simulink model "sf_abstemporal_basic"  (R2017b)
settings: Solver=FixedStepDiscrete  StartTime=0.0  StopTime=10.0  FixedStep=0.1  RelTol=1e-3  EnableMultiTasking=on
settings Model: Creator=The MathWorks, Inc.  LastModifiedBy=The MathWorks, Inc.
settings DataIOCC: LimitDataPoints=on  SaveFormat=Array
settings OptimizationCC: ExpressionDepthLimit=2147483647  LifeSpan=inf
settings DebuggingCC: UnderspecifiedInitializationDetection=Classic  MergeDetectMultiDrivingBlocksExec=none  SolverPrmCheckMsg=warning  FcnCallInpInsideContextMsg=warning  StateNameClashWarn=warning  StrictBusMsg=Warning  SFUnexpectedBacktrackingDiag=warning  SFNoUnconditionalDefaultTransitionDiag=warning  SFExecutionAtInitializationDiag=none
settings HardwareCC: ProdBitPerPointer=32  ProdBitPerSizeT=32  ProdBitPerPtrDiffT=32  ProdLargestAtomicFloat=None  ProdIntDivRoundTo=Undefined  ProdEndianess=Unspecified  ProdWordSize=32  ProdHWDeviceType=32-bit Generic
settings ModelReferenceCC: PropagateSignalLabelsOutOfModel=off
settings SFSimCC: SimParseCustomCode=off
settings CodeAppCC: StateflowObjectComments=on
settings GRTTargetCC: TargetLangStandard=C89/C90 (ANSI)  GeneratePreprocessorConditionals=Disable all  CombineOutputUpdateFcns=off  GRTInterface=on
settings ConfigComp: CovMetricSettings=dw  CovHtmlReporting=on  CovSaveCumulativeToWorkspaceVar=on  CovSaveSingleToWorkspaceVar=on  CovExternalEMLEnable=off  CovSFcnEnable=off

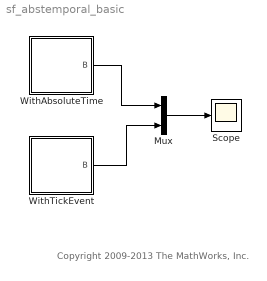
== system sf_abstemporal_basic ==
  note: Copyright 2009-2013 The MathWorks, Inc.
  Mux : Mux  Inputs=2
  Scope : Scope
  WithAbsoluteTime : Stateflow chart  TreatAsAtomicUnit=on
  WithTickEvent : Stateflow chart  TreatAsAtomicUnit=on
  wires:
  WithTickEvent/1(" B") -> Mux/2
  Mux/1 -> Scope/1
  WithAbsoluteTime/1(" B") -> Mux/1

== stateflow chart sf_abstemporal_basic/WithAbsoluteTime ==
  state A
  state B
  (default) -> A
  A -> B : after(3,sec)
  data: B output boolean

== stateflow chart sf_abstemporal_basic/WithTickEvent ==
  state A
  state B
  (default) -> A
  A -> B : after(30,tick)
  data: B output boolean
